simulink model "BLDC_PID080927"  (Simulink 7.1)
settings: Solver=ode4  StartTime=0  StopTime=0.4  FixedStep=Ts  MaxStep=1e-6  RelTol=1e-6  AbsTol=1e-6
PreLoadFcn:
  | assignin('base','Ts',[5e-6])
undefined symbols (not defined in the file): Ts
libraries: powerlib x17, simulink x6, powerlib_extras x1
Description:
  | This demonstration illustrates use of the BLDC in a closed-loop
  | speed and voltage control on a 1 kW, 3000 rpm industrial motor
settings Model: Creator=Olivier Tremblay  LastModifiedBy=Administrator  ExtModeAutoUpdateStatusClock=off
settings DataIOCC: SignalLoggingName=sigsOut
settings OptimizationCC: InlineInvariantSignals=on
settings DebuggingCC: SignalResolutionControl=TryResolveAllWithWarning  SolverPrmCheckMsg=none  MultiTaskDSMMsg=warning  MultiTaskCondExecSysMsg=none  StrictBusMsg=None
settings HardwareCC: TargetUnknown=on
settings RTWCC: IncludeERTFirstTime=on

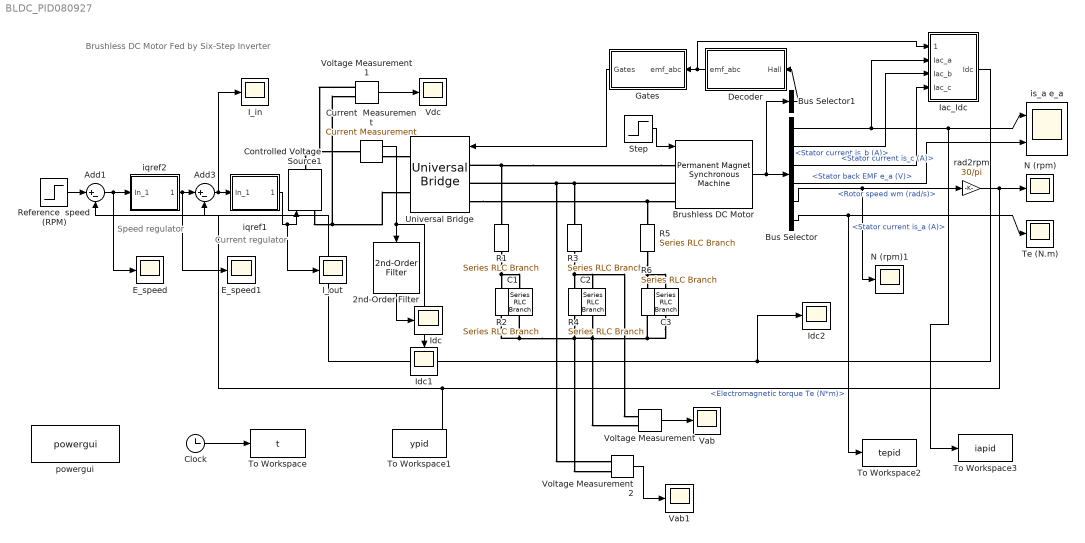
== system BLDC_PID080927 ==
  note: Brushless DC Motor Fed by Six-Step Inverter
  note: Current
      | regulator
  note: Speed
      | regulator
  2nd-Order Filter : powerlib_extras/Control  Blocks/2nd-Order Filter  Orientation=down  DialogController=POWERSYS.PowerSysDialog  SystemSampleTime=-1  FilterType=Lowpass  Fo=50  Zeta=0.707  Initialize=off  Vac_Init=[1 45 60]  Vdc_Init=-0.5  PlotResponse=off  param1=[1 500 1]
  Add1 : Sum  Inputs=|+-  OutDataType=sfix(16)  OutScaling=2^-10
  Add3 : Sum  Inputs=|+-  OutDataType=sfix(16)  OutScaling=2^-10
  Brushless DC Motor : powerlib/Machines/Permanent Magnet Synchronous Machine  DialogController=POWERSYS.PowerSysDialog  SystemSampleTime=-1  FluxDistribution=Trapezoidal  MechanicalLoad=Torque Tm  PresetModel=No  ShowDetailedParameters=on  Resistance=0.6  Inductance=0.205e-3  dqInductances=[8.5e-3, 8.5e-3]  MachineConstant=Torque Constant (N.m / A_peak)  Flux=0.0015958  VoltageCst=2.6738  TorqueCst=0.025533  Flat=120  Mechanical="[9.25e-6, 1e-9,  8]"  PolePairs=8  InitialConditions=[0,0, 0,0]  TsPowergui=0  TsBlock=-1
  Bus Selector : BusSelector  OutputSignals=Stator current is_a (A),Stator current is_b (A),Stator current is_c (A),Stator back EMF e_a (V),Rotor speed wm (rad/s),Electromagnetic torque Te (N*m)
  Bus Selector1 : BusSelector  OutputSignals=Hall effect signal h_a,Hall effect signal h_b,Hall effect signal h_c  OutputAsBus=on
  C1 : powerlib/Elements/Series RLC Branch  Orientation=down  DialogController=POWERSYS.PowerSysDialog  PhysicalDomain=powersysdomain  SubClassName=unknown  LeftPortType=p1  RightPortType=p1  LConnTagsString=__new0  RConnTagsString=__new0  BranchType=C  Resistance=1  Inductance=1e-3  SetiL0=off  InitialCurrent=0  Capacitance=1e-6  Setx0=off  InitialVoltage=0  Measurements=None
  C2 : powerlib/Elements/Series RLC Branch  Orientation=down  DialogController=POWERSYS.PowerSysDialog  PhysicalDomain=powersysdomain  SubClassName=unknown  LeftPortType=p1  RightPortType=p1  LConnTagsString=__new0  RConnTagsString=__new0  BranchType=C  Resistance=1  Inductance=1e-3  SetiL0=off  InitialCurrent=0  Capacitance=1e-4  Setx0=off  InitialVoltage=0  Measurements=None
  C3 : powerlib/Elements/Series RLC Branch  Orientation=down  DialogController=POWERSYS.PowerSysDialog  PhysicalDomain=powersysdomain  SubClassName=unknown  LeftPortType=p1  RightPortType=p1  LConnTagsString=__new0  RConnTagsString=__new0  BranchType=C  Resistance=1  Inductance=1e-3  SetiL0=off  InitialCurrent=0  Capacitance=1e-6  Setx0=off  InitialVoltage=0  Measurements=None
  Clock : Clock
      settings: Decimation=10
  Controlled Voltage Source1 : powerlib/Electrical Sources/Controlled Voltage Source  Orientation=up  DialogController=POWERSYS.PowerSysDialog  SystemSampleTime=-1  Initialize=on  Source_Type=AC  Amplitude=12  Phase=0  Frequency=0  Measurements=None
  Current  Measurement : powerlib/Measurements/Current Measurement  DialogController=POWERSYS.PowerSysDialog  SystemSampleTime=-1  PhasorSimulation=off  OutputType=Complex  PSBequivalent=0
  Decoder : Subsystem  Orientation=left
  E_speed : Scope
      settings: TimeRange=0.2  YMin=0  YMax=500  DataFormat=Structure
  E_speed1 : Scope
      settings: TimeRange=0.2  YMin=0  YMax=500  SaveName=ScopeData9  DataFormat=Structure
  Gates : Subsystem  Orientation=left
  I_in : Scope
      settings: TimeRange=0.35  YMin=-0.4  YMax=1.6  SaveName=ScopeData2  DataFormat=Structure
  I_out : Scope
      settings: TimeRange=0.35  YMin=4.55  YMax=5.6  SaveName=ScopeData5  DataFormat=Structure
  Iac_Idc : Subsystem
  Idc : Scope
      settings: TimeRange=0.35  YMin=-0.4  YMax=1.6  DataFormat=Structure
  Idc1 : Scope
      settings: Orientation=down  TimeRange=0.35  YMin=-0.4  YMax=1.6  SaveName=ScopeData7  DataFormat=Structure
  Idc2 : Scope
      settings: TimeRange=0.35  YMin=-0.4  YMax=1.6  SaveName=ScopeData6  DataFormat=Structure
  N (rpm) : Scope
      settings: TimeRange=0.4  YMin=0  YMax=1200  SaveName=N
  N (rpm)1 : Scope
      settings: TimeRange=0.4  YMin=0  YMax=1200  SaveName=N2
  R{1..2,5..6} (4 alike) : powerlib/Elements/Series RLC Branch  Orientation=down  DialogController=POWERSYS.PowerSysDialog  PhysicalDomain=powersysdomain  SubClassName=unknown  LeftPortType=p1  RightPortType=p1  LConnTagsString=__new0  RConnTagsString=__new0  BranchType=R  Resistance=1  Inductance=1e-3  SetiL0=off  InitialCurrent=0  Capacitance=1e-6  Setx0=off  InitialVoltage=0  Measurements=None
  R3 : powerlib/Elements/Series RLC Branch  Orientation=down  DialogController=POWERSYS.PowerSysDialog  PhysicalDomain=powersysdomain  SubClassName=unknown  LeftPortType=p1  RightPortType=p1  LConnTagsString=__new0  RConnTagsString=__new0  BranchType=R  Resistance=2  Inductance=1e-3  SetiL0=off  InitialCurrent=0  Capacitance=1e-6  Setx0=off  InitialVoltage=0  Measurements=None
  R4 : powerlib/Elements/Series RLC Branch  Orientation=down  DialogController=POWERSYS.PowerSysDialog  PhysicalDomain=powersysdomain  SubClassName=unknown  LeftPortType=p1  RightPortType=p1  LConnTagsString=__new0  RConnTagsString=__new0  BranchType=R  Resistance=2  Inductance=1e-3  SetiL0=off  InitialCurrent=0  Capacitance=1e-6  Setx0=off  InitialVoltage=0  Measurements=None
  Reference  speed (RPM) : Step  Time=.2  Before=1000  After=2000  SampleTime=0
  Step : Step  Time=.1  After=0.03  SampleTime=0
  Te (N.m) : Scope
      settings: TimeRange=0.2  YMin=0.006  YMax=0.0125  SaveName=N1
  To Workspace : ToWorkspace  VariableName=t  SampleTime=-1  SaveFormat=Array
  To Workspace1 : ToWorkspace  VariableName=ypid  SampleTime=-1  SaveFormat=Array
  To Workspace2 : ToWorkspace  VariableName=tepid  SampleTime=-1  SaveFormat=Array
  To Workspace3 : ToWorkspace  VariableName=iapid  SampleTime=-1  SaveFormat=Array
  Universal Bridge : powerlib/Power Electronics/Universal Bridge  Orientation=left  DialogController=POWERSYS.PowerSysDialog  SystemSampleTime=-1  Arms=3  SnubberResistance=5000  SnubberCapacitance=1e-6  Device=MOSFET / Diodes  Ron=1e-3  Lon=0  ForwardVoltages="[  0  0  ]"  ForwardVoltage=0  GTOparameters=[ 10e-6 , 20e-6 ]  IGBTparameters=[ 1e-6 , 2e-6 ]  Measurements=Device currents  converterType=Rectifier
  Vab : Scope
      settings: TimeRange=0.06  YMin=-10000  YMax=10000  SaveName=ScopeData4  DataFormat=Structure
  Vab1 : Scope
      settings: TimeRange=0.06  YMin=-10000  YMax=10000  SaveName=ScopeData8  DataFormat=Structure
  Vdc : Scope
      settings: TimeRange=0.2  YMin=3.75  YMax=7.5  SaveName=ScopeData3  DataFormat=Structure
  Voltage Measurement : powerlib/Measurements/Voltage Measurement  DialogController=POWERSYS.PowerSysDialog  SystemSampleTime=-1  PhasorSimulation=off  OutputType=Complex  PSBequivalent=0
  Voltage Measurement1 : powerlib/Measurements/Voltage Measurement  DialogController=POWERSYS.PowerSysDialog  SystemSampleTime=-1  PhasorSimulation=off  OutputType=Complex  PSBequivalent=0
  Voltage Measurement2 : powerlib/Measurements/Voltage Measurement  DialogController=POWERSYS.PowerSysDialog  SystemSampleTime=-1  PhasorSimulation=off  OutputType=Complex  PSBequivalent=0
  iqref1 : Subsystem  mask(PI Controller){@1=5, @2=8, @3=[-12, 12]}
      mask prompts: @1 "Integral"; @2 "Proportional:"; @3 "Minimum and maximum outputs:"
      mask init:
      | I=@1;P=@2;sat=@3;min=sat(1);max=sat(2);
      mask Display: disp('PI')
  iqref2 : Subsystem  mask(PI Controller){@1=0.15, @2=0.5, @3=[-2.3, 2.3]}
      mask prompts: @1 "Integral"; @2 "Proportional:"; @3 "Minimum and maximum outputs:"
      mask init:
      | I=@1;P=@2;sat=@3;min=sat(1);max=sat(2);
      mask Display: disp('PI')
  is_a e_a : Scope  NumInputPorts=2
      settings: TimeRange=0.2  YMin=-15~-250  YMax=20~250  SaveName=IE
  powergui : powerlib/powergui  Priority=2  SystemSampleTime=-1  SimulationMode=Discrete  SampleTime=Ts  frequency=60  SPID=off  SwTol=0  Interpol=off  x0status=blocks  echomessages=off  HookPort=off  FunctionMessages=off  EnableUseOfTLC=off  RestoreLinks=warning  frequencyindice=0  Frange=[0:2:500]  Ylog=off  Xlog=on  ShowGrid=off  save=off  variable=ZData  ZoomFFT=on  StartTime=0.0  cycles=1  DisplayStyle=1  fundamental=60  FreqAxis=off  MaxFrequency=1000  frequencyindicesteady=1  RmsSteady=1  display=off  Ts=0  methode=off
  rad2rpm : Gain  Gain=30/pi  ParameterDataType=sfix(16)  ParameterScaling=2^0  OutDataType=sfix(16)  OutScaling=2^0
  wires:
  Step/1 -> Brushless DC Motor/1
  iqref1/1(Out_1) -> Controlled Voltage Source1/1, I_out/1
  Add3/1 -> I_in/1, iqref1/1(In_1)
  Gates/1(Gates) -> Universal Bridge/1
  Decoder/1(emf_abc) -> Gates/1("emf_abc "), Iac_Idc/1(switch)
  rad2rpm/1 -> N (rpm)/1, Add1/2, To Workspace1/1
  Voltage Measurement/1 -> Vab/1
  Voltage Measurement1/1 -> Vdc/1
  Bus Selector/1 -> Iac_Idc/2(Iac_a), is_a e_a/1, To Workspace3/1  "<Stator current is_a (A)>"
  Brushless DC Motor/1 -> Bus Selector/1, Bus Selector1/1
  Bus Selector1/1 -> Decoder/1("Hall ")
  Bus Selector/4 -> is_a e_a/2  "<Stator back EMF e_a (V)>"
  Bus Selector/5 -> rad2rpm/1, N (rpm)1/1  "<Rotor speed wm (rad/s)>"
  Bus Selector/6 -> Te (N.m)/1, To Workspace2/1  "<Electromagnetic torque Te (N*m)>"
  Current  Measurement/1 -> 2nd-Order Filter/1, Idc1/1
  Reference  speed (RPM)/1 -> Add1/1
  2nd-Order Filter/1 -> Idc/1
  Bus Selector/2 -> Iac_Idc/3(Iac_b)  "<Stator current is_b (A)>"
  Iac_Idc/1(Idc) -> Idc2/1, Add3/2
  iqref2/1(Out_1) -> Add3/1, E_speed1/1
  Bus Selector/3 -> Iac_Idc/4(Iac_c)  "<Stator current is_c (A)>"
  Add1/1 -> E_speed/1, iqref2/1(In_1)
  Clock/1 -> To Workspace/1
  Voltage Measurement2/1 -> Vab1/1
  connections:
  Brushless DC Motor/LConn1 -- Universal Bridge/LConn1 -- R1/LConn1
  Brushless DC Motor/LConn2 -- R3/LConn1 -- Universal Bridge/LConn2 -- Voltage Measurement2/LConn1
  Universal Bridge/LConn3 -- Brushless DC Motor/LConn3 -- R5/LConn1
  Controlled Voltage Source1/RConn1 -- Voltage Measurement1/LConn1 -- Current  Measurement/LConn1
  Controlled Voltage Source1/LConn1 -- Universal Bridge/RConn2 -- Voltage Measurement1/LConn2
  Current  Measurement/RConn1 -- Universal Bridge/RConn1
  R1/RConn1 -- R2/LConn1 -- C1/LConn1
  C2/LConn1 -- R3/RConn1 -- R4/LConn1 -- Voltage Measurement/LConn1
  C3/LConn1 -- R5/RConn1 -- R6/LConn1
  C1/RConn1 -- R2/RConn1 -- C2/RConn1 -- R6/RConn1 -- C3/RConn1 -- Voltage Measurement/LConn2 -- R4/RConn1 -- Voltage Measurement2/LConn2

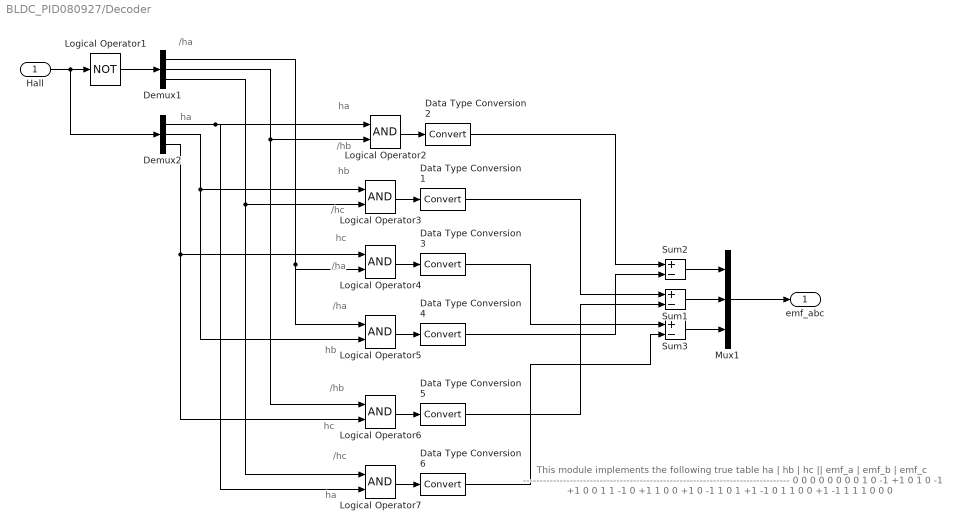
== system BLDC_PID080927/Decoder ==
  note: /ha
  note: ha
  note: ha
  note: /hb
  note: hb
  note: /hc
  note: hc
  note: /ha
  note: /ha
  note: hb
  note: /hb
  note: hc
  note: /hc
  note: ha
  note: This module implements the following true table
      |
      |    ha   |   hb   |   hc   ||   emf_a   |   emf_b   |   emf_c
      |     --------------------------------------------------------------------------------
      | 0          0         0          0               0               0
      | 0          0         1          0               -1               +1
      | 0          1         0          -1              +1                0
      | 0          1         1          -1               0               +1
      | 1          0         0         +1               0               -1
      | 1          0         1         +1              -1                0
      | 1          1         0          0              +1               -1
      | 1          1         1          0               0                0
  "Hall " : Inport  OutDataType=sfix(16)  OutScaling=2^0
  Data Type Conversion{1..6} (6 alike) : DataTypeConversion  OutDataType=sfix(16)  OutScaling=2^0
  Demux1 : Demux  Outputs=3
  Demux2 : Demux  Outputs=3
  Logical Operator1 : Logic  Operator=NOT  AllPortsSameDT=off  OutDataTypeMode=boolean  OutDataTypeStr=boolean
  Logical Operator{2..7} (6 alike) : Logic  AllPortsSameDT=off  OutDataTypeMode=boolean  OutDataTypeStr=boolean
  Mux1 : Mux  Inputs=3
  Sum1 : Sum  Inputs=+-  OutDataTypeMode=double  OutDataType=sfix(16)  OutScaling=2^0  OutDataTypeStr=double
  Sum2 : Sum  Inputs=+-  OutDataTypeMode=double  OutDataType=sfix(16)  OutScaling=2^0  OutDataTypeStr=double
  Sum3 : Sum  Inputs=+-  OutDataTypeMode=double  OutDataType=sfix(16)  OutScaling=2^0  OutDataTypeStr=double
  emf_abc : Outport  OutDataType=sfix(16)  OutScaling=2^0
  wires:
  "Hall "/1 -> Logical Operator1/1, Demux2/1
  Logical Operator1/1 -> Demux1/1
  Demux2/3 -> Logical Operator4/1, Logical Operator6/2
  Demux2/2 -> Logical Operator3/1, Logical Operator5/2
  Demux2/1 -> Logical Operator2/1, Logical Operator7/2
  Demux1/3 -> Logical Operator3/2, Logical Operator7/1
  Demux1/2 -> Logical Operator2/2, Logical Operator6/1
  Demux1/1 -> Logical Operator4/2, Logical Operator5/1
  Logical Operator2/1 -> Data Type Conversion2/1
  Sum2/1 -> Mux1/1
  Sum1/1 -> Mux1/2
  Sum3/1 -> Mux1/3
  Mux1/1 -> emf_abc/1
  Logical Operator3/1 -> Data Type Conversion1/1
  Logical Operator4/1 -> Data Type Conversion3/1
  Logical Operator5/1 -> Data Type Conversion4/1
  Logical Operator6/1 -> Data Type Conversion5/1
  Logical Operator7/1 -> Data Type Conversion6/1
  Data Type Conversion2/1 -> Sum2/1
  Data Type Conversion4/1 -> Sum2/2
  Data Type Conversion1/1 -> Sum1/1
  Data Type Conversion5/1 -> Sum1/2
  Data Type Conversion3/1 -> Sum3/1
  Data Type Conversion6/1 -> Sum3/2

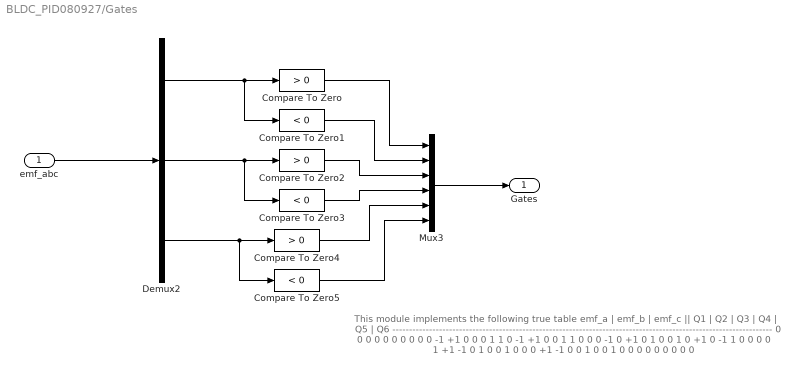
== system BLDC_PID080927/Gates ==
  note: This module implements the following true table
      |
      |    emf_a   |   emf_b   |   emf_c   ||   Q1   |   Q2   |   Q3   |   Q4   |   Q5   |   Q6
      |     ------------------------------------------------------------------------------------------------------------------
      |       0              0                0            0          0          0           0        0        0
      |       0               -1              +1          0          0          0           1        1        0
      |     -1              +1                0          0          1          1           0        0        0
      |     -1               0               +1          0          1         0           0        1        0
      |    +1               0                -1          1          0          0           0        0        1
      |    +1              -1                0           1          0          0           1        0        0
      |      0              +1               -1           0          0          1           0        0        1
      |     0              0                0             0          0          0           0        0        0
  "emf_abc " : Inport  OutDataType=sfix(16)  OutScaling=2^0
  Compare To Zero : simulink/Logic and Bit Operations/Compare To Zero  SystemSampleTime=-1  relop=>  LogicOutDataTypeMode=boolean  ZeroCross=off
  Compare To Zero1 : simulink/Logic and Bit Operations/Compare To Zero  SystemSampleTime=-1  relop=<  LogicOutDataTypeMode=boolean  ZeroCross=off
  Compare To Zero2 : simulink/Logic and Bit Operations/Compare To Zero  SystemSampleTime=-1  relop=>  LogicOutDataTypeMode=boolean  ZeroCross=off
  Compare To Zero3 : simulink/Logic and Bit Operations/Compare To Zero  SystemSampleTime=-1  relop=<  LogicOutDataTypeMode=boolean  ZeroCross=off
  Compare To Zero4 : simulink/Logic and Bit Operations/Compare To Zero  SystemSampleTime=-1  relop=>  LogicOutDataTypeMode=boolean  ZeroCross=off
  Compare To Zero5 : simulink/Logic and Bit Operations/Compare To Zero  SystemSampleTime=-1  relop=<  LogicOutDataTypeMode=boolean  ZeroCross=off
  Demux2 : Demux  Outputs=3
  Mux3 : Mux  Inputs=6
  Gates : Outport  OutDataType=sfix(16)  OutScaling=2^0
  wires:
  "emf_abc "/1 -> Demux2/1
  Mux3/1 -> Gates/1
  Demux2/1 -> Compare To Zero/1, Compare To Zero1/1
  Demux2/2 -> Compare To Zero2/1, Compare To Zero3/1
  Demux2/3 -> Compare To Zero4/1, Compare To Zero5/1
  Compare To Zero/1 -> Mux3/1
  Compare To Zero1/1 -> Mux3/2
  Compare To Zero2/1 -> Mux3/3
  Compare To Zero3/1 -> Mux3/4
  Compare To Zero4/1 -> Mux3/5
  Compare To Zero5/1 -> Mux3/6

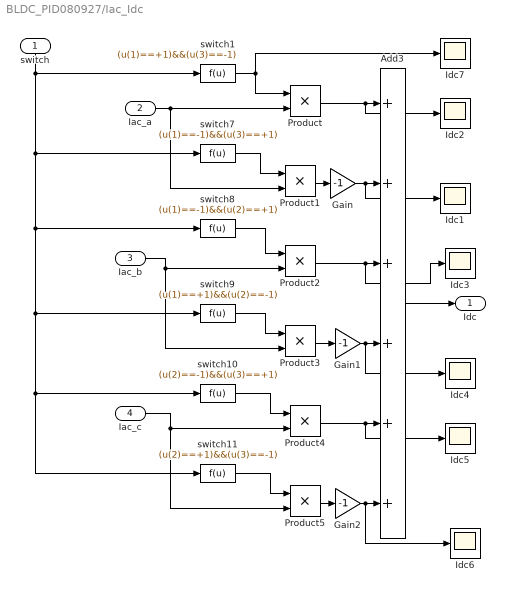
== system BLDC_PID080927/Iac_Idc ==
  switch : Inport  Orientation=down
  Iac_a : Inport  Port=2
  Iac_b : Inport  Port=3
  Iac_c : Inport  Port=4
  Add3 : Sum  Inputs=++++++  OutDataType=sfix(16)  OutScaling=2^-10
  Gain : Gain  Gain=-1  ParameterDataType=sfix(16)  ParameterScaling=2^0  OutDataType=sfix(16)  OutScaling=2^0
  Gain1 : Gain  Gain=-1  ParameterDataType=sfix(16)  ParameterScaling=2^0  OutDataType=sfix(16)  OutScaling=2^0
  Gain2 : Gain  Gain=-1  ParameterDataType=sfix(16)  ParameterScaling=2^0  OutDataType=sfix(16)  OutScaling=2^0
  Idc{1..7} (7 alike) : Scope
      Idc1 settings: TimeRange=0.35  YMin=-0.4  YMax=1.6  SaveName=ScopeData11  DataFormat=Structure
      Idc2 settings: TimeRange=0.35  YMin=-0.4  YMax=1.6  SaveName=ScopeData10  DataFormat=Structure
      Idc3 settings: TimeRange=0.35  YMin=-0.4  YMax=1.6  SaveName=ScopeData12  DataFormat=Structure
      Idc4 settings: TimeRange=0.35  YMin=-0.4  YMax=1.6  SaveName=ScopeData13  DataFormat=Structure
      Idc5 settings: TimeRange=0.35  YMin=-0.4  YMax=1.6  SaveName=ScopeData14  DataFormat=Structure
      Idc6 settings: TimeRange=0.35  YMin=-0.4  YMax=1.6  SaveName=ScopeData15  DataFormat=Structure
      Idc7 settings: TimeRange=0.35  YMin=-0.4  YMax=1.6  SaveName=ScopeData16  DataFormat=Structure
  Product{,1..5} (6 alike) : Product  OutDataType=sfix(16)  OutScaling=2^0  RndMeth=Zero
  switch1 : Fcn  Expr=(u(1)==+1)&&(u(3)==-1)
  switch10 : Fcn  Expr=(u(2)==-1)&&(u(3)==+1)
  switch11 : Fcn  Expr=(u(2)==+1)&&(u(3)==-1)
  switch7 : Fcn  Expr=(u(1)==-1)&&(u(3)==+1)
  switch8 : Fcn  Expr=(u(1)==-1)&&(u(2)==+1)
  switch9 : Fcn  Expr=(u(1)==+1)&&(u(2)==-1)
  Idc : Outport
  wires:
  switch1/1 -> Idc7/1, Product/1
  switch/1 -> switch1/1, switch7/1, switch8/1, switch9/1, switch10/1, switch11/1
  Iac_a/1 -> Product/2, Product1/2
  Iac_b/1 -> Product2/2, Product3/2
  Iac_c/1 -> Product4/2, Product5/2
  switch11/1 -> Product5/1
  Product/1 -> Idc2/1, Add3/1
  Product1/1 -> Gain/1
  Product2/1 -> Add3/3, Idc3/1
  Product3/1 -> Gain1/1
  Product4/1 -> Add3/5, Idc5/1
  Product5/1 -> Gain2/1
  Add3/1 -> Idc/1
  switch7/1 -> Product1/1
  Gain/1 -> Add3/2, Idc1/1
  switch8/1 -> Product2/1
  switch9/1 -> Product3/1
  Gain1/1 -> Idc4/1, Add3/4
  switch10/1 -> Product4/1
  Gain2/1 -> Idc6/1, Add3/6

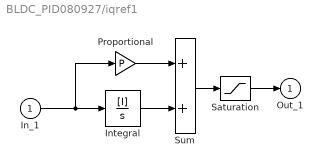
== system BLDC_PID080927/iqref1 ==
  In_1 : Inport  OutDataType=sfix(16)  OutScaling=2^0
  Integral : TransferFcn  Numerator=[I]  Denominator=[1 0]
  Proportional : Gain  Gain=P  ParameterDataType=sfix(16)  ParameterScaling=2^0  OutDataType=sfix(16)  OutScaling=2^0  SaturateOnIntegerOverflow=on  OutDataTypeStr=Inherit: Same as input  ParamDataTypeStr=Inherit: Same as input
  Saturation : Saturate  UpperLimit=max  LowerLimit=min  OutDataType=sfix(16)  OutScaling=2^0
  Sum : Sum  OutDataType=sfix(16)  OutScaling=2^0  SaturateOnIntegerOverflow=on  InputSameDT=on  OutDataTypeStr=Inherit: Same as first input
  Out_1 : Outport  OutDataType=sfix(16)  OutScaling=2^0  InitialOutput=0
  wires:
  Saturation/1 -> Out_1/1
  Sum/1 -> Saturation/1
  Proportional/1 -> Sum/1
  In_1/1 -> Proportional/1, Integral/1
  Integral/1 -> Sum/2

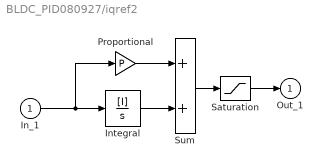
== system BLDC_PID080927/iqref2 ==
  In_1 : Inport  OutDataType=sfix(16)  OutScaling=2^0
  Integral : TransferFcn  Numerator=[I]  Denominator=[1 0]
  Proportional : Gain  Gain=P  ParameterDataType=sfix(16)  ParameterScaling=2^0  OutDataType=sfix(16)  OutScaling=2^0  SaturateOnIntegerOverflow=on  OutDataTypeStr=Inherit: Same as input  ParamDataTypeStr=Inherit: Same as input
  Saturation : Saturate  UpperLimit=max  LowerLimit=min  OutDataType=sfix(16)  OutScaling=2^0
  Sum : Sum  OutDataType=sfix(16)  OutScaling=2^0  SaturateOnIntegerOverflow=on  InputSameDT=on  OutDataTypeStr=Inherit: Same as first input
  Out_1 : Outport  OutDataType=sfix(16)  OutScaling=2^0  InitialOutput=0
  wires:
  Integral/1 -> Sum/2
  In_1/1 -> Integral/1, Proportional/1
  Proportional/1 -> Sum/1
  Sum/1 -> Saturation/1
  Saturation/1 -> Out_1/1
